simulink model "Prob_1"  (R2020b)
settings: Solver=VariableStepAuto  StartTime=0.0  StopTime=10.0  RelTol=1e-3
undefined symbols (not defined in the file): b, k1, k12, m1, m2
settings Model: Creator=kshir  LastModifiedBy=kshir

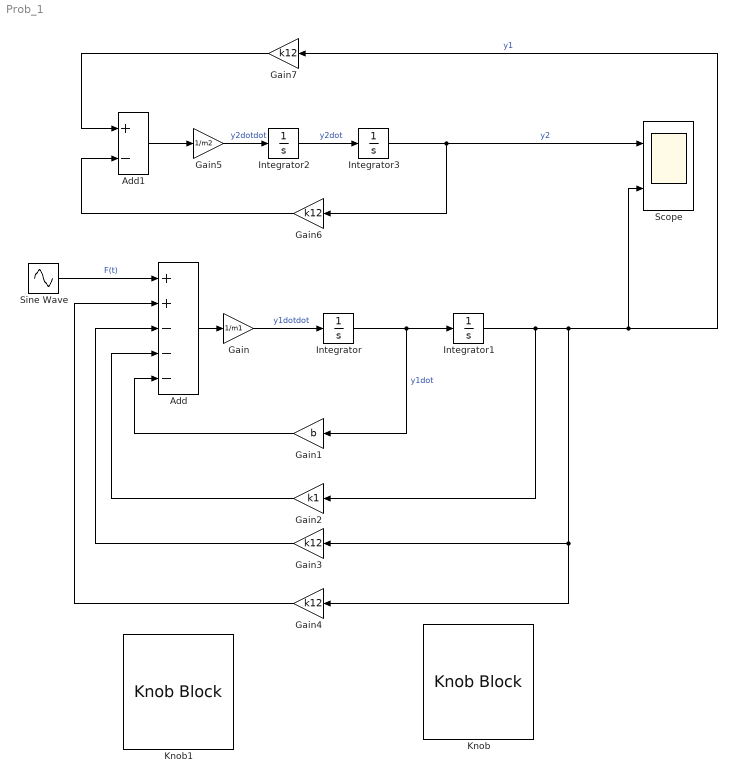
== system Prob_1 ==
  Add : Sum  Inputs=++---
  Add1 : Sum  Inputs=+-
  Gain : Gain  Gain=1/m1
  Gain1 : Gain  Gain=b
  Gain2 : Gain  Gain=k1
  Gain{3..4,6..7} (4 alike) : Gain  Gain=k12
  Gain5 : Gain  Gain=1/m2
  Integrator{,1..3} (4 alike) : Integrator
  Knob : KnobBlock  ScaleMin=-500  ScaleMax=10000
  Knob1 : KnobBlock
  Scope : Scope  NumInputPorts=2
  Sine Wave : Sin  Amplitude=2  Frequency=10  SampleTime=0
  wires:
  Sine Wave/1 -> Add/1  "F(t)"
  Add/1 -> Gain/1
  Gain/1 -> Integrator/1  "y1dotdot"
  Integrator/1 -> Gain1/1, Integrator1/1  "y1dot"
  Integrator1/1 -> Gain2/1, Scope/2, Gain7/1, Gain3/1, Gain4/1  "y1"
  Gain1/1 -> Add/5
  Gain2/1 -> Add/4
  Gain3/1 -> Add/3
  Gain4/1 -> Add/2
  Add1/1 -> Gain5/1
  Gain5/1 -> Integrator2/1  "y2dotdot"
  Integrator2/1 -> Integrator3/1  "y2dot"
  Integrator3/1 -> Gain6/1, Scope/1  "y2"
  Gain6/1 -> Add1/2
  Gain7/1 -> Add1/1
